simulink model "Sistema_real_NL_Din_residual"  (R2023b)
settings: Solver=VariableStepAuto  StartTime=0.0  StopTime=10.0  RelTol=1e-3
values from neighbouring files (symbols this model uses):
  alpha_cu = 3.9*10^-3    (= 0.0039)    [polos_y_ceros.m]    (also in var1.m)
  b_eq = b_m + b_l/(r^2)    (= 2.19444444444e-05)    [polos_y_ceros.m]    (also in var1.m)
  C_ts = 0.818    [polos_y_ceros.m]    (also in var1.m)
  J_eq = J_m + J_l/(r^2)    (= 1.97847222222e-05)    [polos_y_ceros.m]    (also in var1.m = 4.58263888889e-05)
  k_l = m * L_cm + m_l * L_l    (= 0.25)    [polos_y_ceros.m]    (also in var1.m = 1)
  L_d = 6.6 * 10^(-3)    (= 0.0066)    [polos_y_ceros.m]    (also in var1.m)
  L_ls = 0.8 * 10^(-3)    (= 0.0008)    [polos_y_ceros.m]    (also in var1.m)
  L_q = 5.8 * 10^(-3)    (= 0.0058)    [polos_y_ceros.m]    (also in var1.m)
  lambda_m = 0.016    [polos_y_ceros.m]    (also in var1.m)
  P_p = 3    [polos_y_ceros.m]    (also in var1.m)
  r = 120/1    (= 120)    [polos_y_ceros.m]    (also in var1.m)
  R_sREF = 1.02    [polos_y_ceros.m]    (also in var1.m)
  R_ts_amb = 146.7    [polos_y_ceros.m]    (also in var1.m)
undefined symbols (not defined in the file or in its folder): magnitude
settings Model: Creator=tomas  LastModifiedBy=tomas

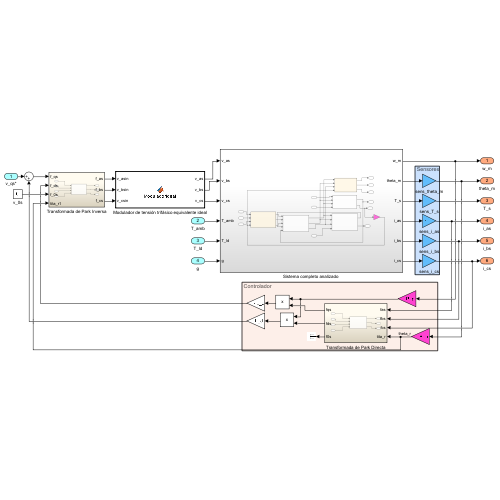
[thumbnail: Simulink's stored preview of the top-level diagram]
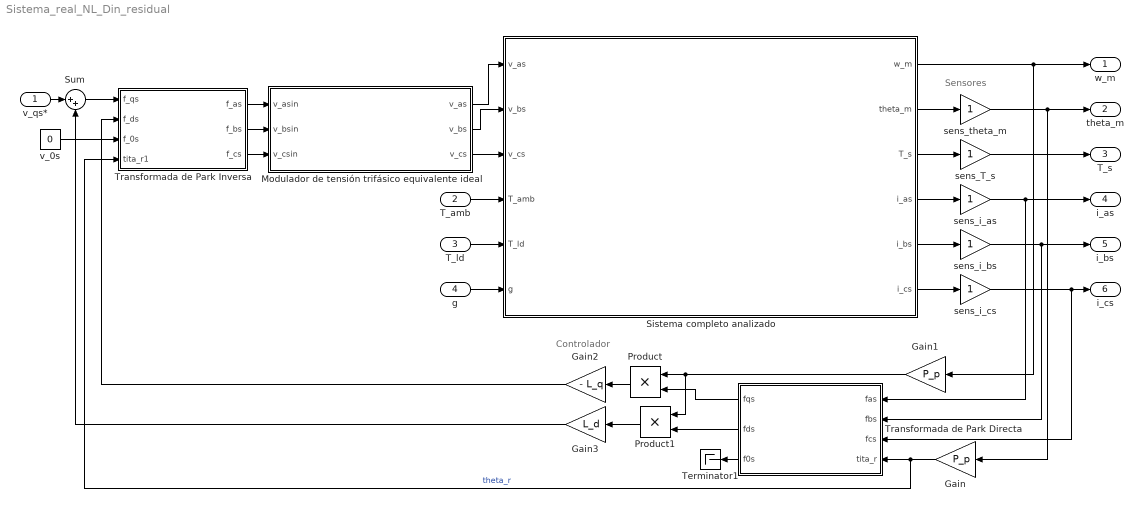
== system Sistema_real_NL_Din_residual ==
  note: Controlador
  note: Sensores
  v_qs* : Inport
  T_amb : Inport  Port=2
  T_ld : Inport  Port=3
  g : Inport  Port=4
  Gain : Gain  Gain=P_p
  Gain1 : Gain  Gain=P_p
  Gain2 : Gain  Gain=- L_q
  Gain3 : Gain  Gain=L_d
  Modulador de tensión trifásico equivalente ideal : MATLAB Function  TreatAsAtomicUnit=on
  Product : Product
  Product1 : Product
  "Sistema completo analizado " : Subsystem
  Sum : Sum  Inputs=|++
  Terminator1 : Terminator
  Transformada de Park Directa : Subsystem
  Transformada de Park Inversa : Subsystem
  sens_T_s : Gain
  sens_i_as : Gain
  sens_i_bs : Gain
  sens_i_cs : Gain
  sens_theta_m : Gain
  v_0s : Constant  Value=0
  w_m : Outport
  theta_m : Outport  Port=2
  T_s : Outport  Port=3
  i_as : Outport  Port=4
  i_bs : Outport  Port=5
  i_cs : Outport  Port=6
  wires:
  Transformada de Park Directa/3(f0s) -> Terminator1/1
  Transformada de Park Directa/2(fds) -> Product1/2
  T_ld/1 -> "Sistema completo analizado "/5(T_ld)
  Transformada de Park Inversa/3(f_cs) -> Modulador de tensión trifásico equivalente ideal/3(v_csin)
  Transformada de Park Inversa/1(f_as) -> Modulador de tensión trifásico equivalente ideal/1(v_asin)
  Transformada de Park Inversa/2(f_bs) -> Modulador de tensión trifásico equivalente ideal/2(v_bsin)
  "Sistema completo analizado "/6(i_cs) -> sens_i_cs/1
  Product/1 -> Gain2/1
  sens_i_bs/1 -> Transformada de Park Directa/2(fbs), i_bs/1
  Modulador de tensión trifásico equivalente ideal/1(v_as) -> "Sistema completo analizado "/1(v_as)
  v_0s/1 -> Transformada de Park Inversa/3(f_0s)
  "Sistema completo analizado "/4(i_as) -> sens_i_as/1
  Gain/1 -> Transformada de Park Inversa/4(tita_r1), Transformada de Park Directa/4(tita_r)  "theta_r"
  Transformada de Park Directa/1(fqs) -> Product/2
  sens_T_s/1 -> T_s/1
  "Sistema completo analizado "/3(T_s) -> sens_T_s/1
  "Sistema completo analizado "/2(theta_m) -> sens_theta_m/1
  "Sistema completo analizado "/5(i_bs) -> sens_i_bs/1
  Modulador de tensión trifásico equivalente ideal/3(v_cs) -> "Sistema completo analizado "/3(v_cs)
  Modulador de tensión trifásico equivalente ideal/2(v_bs) -> "Sistema completo analizado "/2(v_bs)
  sens_i_cs/1 -> Transformada de Park Directa/3(fcs), i_cs/1
  T_amb/1 -> "Sistema completo analizado "/4(T_amb)
  Gain2/1 -> Transformada de Park Inversa/2(f_ds)
  sens_i_as/1 -> Transformada de Park Directa/1(fas), i_as/1
  "Sistema completo analizado "/1(w_m) -> Gain1/1, w_m/1
  Gain1/1 -> Product1/1, Product/1
  sens_theta_m/1 -> Gain/1, theta_m/1
  Product1/1 -> Gain3/1
  Gain3/1 -> Sum/2
  v_qs*/1 -> Sum/1
  Sum/1 -> Transformada de Park Inversa/1(f_qs)
  g/1 -> "Sistema completo analizado "/6(g)

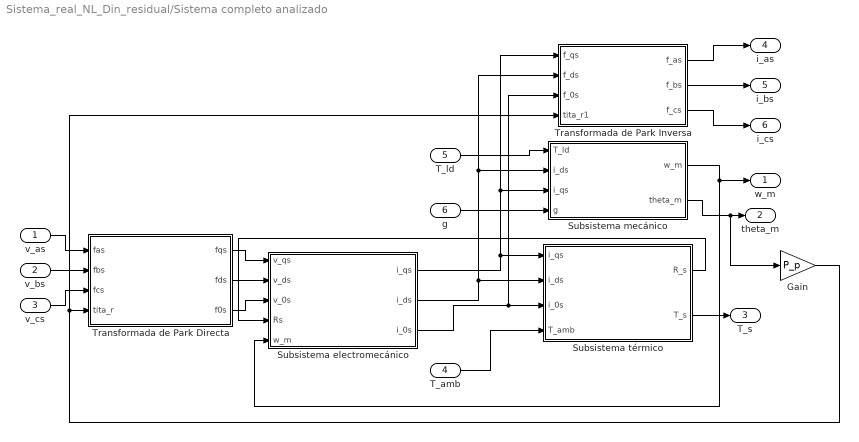
== system Sistema_real_NL_Din_residual/Sistema completo analizado  ==
  v_as : Inport
  v_bs : Inport  Port=2
  v_cs : Inport  Port=3
  T_amb : Inport  Port=4
  T_ld : Inport  Port=5
  g : Inport  Port=6
  Gain : Gain  Gain=P_p
  Subsistema electromecánico : Subsystem
  Subsistema mecánico : Subsystem
  Subsistema térmico : Subsystem
  Transformada de Park Directa : Subsystem
  Transformada de Park Inversa : Subsystem
  w_m : Outport
  theta_m : Outport  Port=2
  T_s : Outport  Port=3
  i_as : Outport  Port=4
  i_bs : Outport  Port=5
  i_cs : Outport  Port=6
  wires:
  Transformada de Park Inversa/3(f_cs) -> i_cs/1
  Subsistema mecánico/1(w_m) -> w_m/1, Subsistema electromecánico/5(w_m)
  Subsistema electromecánico/3(i_0s) -> Transformada de Park Inversa/3(f_0s), Subsistema térmico/3(i_0s)
  Transformada de Park Directa/1(fqs) -> Subsistema electromecánico/1(v_qs)
  Subsistema térmico/2(T_s) -> T_s/1
  Transformada de Park Directa/3(f0s) -> Subsistema electromecánico/3(v_0s)
  Subsistema electromecánico/2(i_ds) -> Transformada de Park Inversa/2(f_ds), Subsistema mecánico/2(i_ds), Subsistema térmico/2(i_ds)
  Gain/1 -> Transformada de Park Inversa/4(tita_r1), Transformada de Park Directa/4(tita_r)
  T_ld/1 -> Subsistema mecánico/1(T_ld)
  Transformada de Park Directa/2(fds) -> Subsistema electromecánico/2(v_ds)
  Transformada de Park Inversa/2(f_bs) -> i_bs/1
  v_bs/1 -> Transformada de Park Directa/2(fbs)
  T_amb/1 -> Subsistema térmico/4(T_amb)
  Transformada de Park Inversa/1(f_as) -> i_as/1
  v_as/1 -> Transformada de Park Directa/1(fas)
  Subsistema mecánico/2(theta_m) -> Gain/1, theta_m/1
  v_cs/1 -> Transformada de Park Directa/3(fcs)
  Subsistema electromecánico/1(i_qs) -> Transformada de Park Inversa/1(f_qs), Subsistema mecánico/3(i_qs), Subsistema térmico/1(i_qs)
  Subsistema térmico/1(R_s) -> Subsistema electromecánico/4(Rs)
  g/1 -> Subsistema mecánico/4(g)

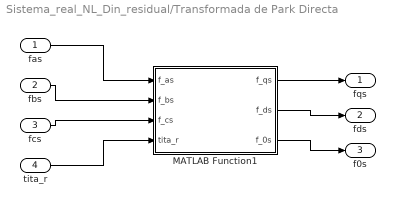
== system Sistema_real_NL_Din_residual/Transformada de Park Directa ==
  fas : Inport
  fbs : Inport  Port=2
  fcs : Inport  Port=3
  tita_r : Inport  Port=4
  MATLAB Function1 : MATLAB Function  TreatAsAtomicUnit=on
  fqs : Outport
  fds : Outport  Port=2
  f0s : Outport  Port=3
  wires:
  fas/1 -> MATLAB Function1/1(f_as)
  MATLAB Function1/3(f_0s) -> f0s/1
  MATLAB Function1/2(f_ds) -> fds/1
  fbs/1 -> MATLAB Function1/2(f_bs)
  fcs/1 -> MATLAB Function1/3(f_cs)
  tita_r/1 -> MATLAB Function1/4(tita_r)
  MATLAB Function1/1(f_qs) -> fqs/1

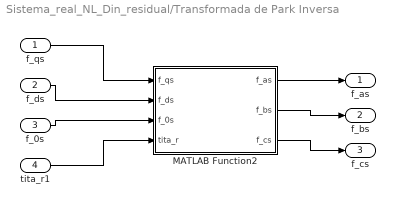
== system Sistema_real_NL_Din_residual/Transformada de Park Inversa ==
  f_qs : Inport
  f_ds : Inport  Port=2
  f_0s : Inport  Port=3
  tita_r1 : Inport  Port=4
  MATLAB Function2 : MATLAB Function  TreatAsAtomicUnit=on
  f_as : Outport
  f_bs : Outport  Port=2
  f_cs : Outport  Port=3
  wires:
  tita_r1/1 -> MATLAB Function2/4(tita_r)
  MATLAB Function2/2(f_bs) -> f_bs/1
  MATLAB Function2/1(f_as) -> f_as/1
  f_ds/1 -> MATLAB Function2/2(f_ds)
  MATLAB Function2/3(f_cs) -> f_cs/1
  f_0s/1 -> MATLAB Function2/3(f_0s)
  f_qs/1 -> MATLAB Function2/1(f_qs)

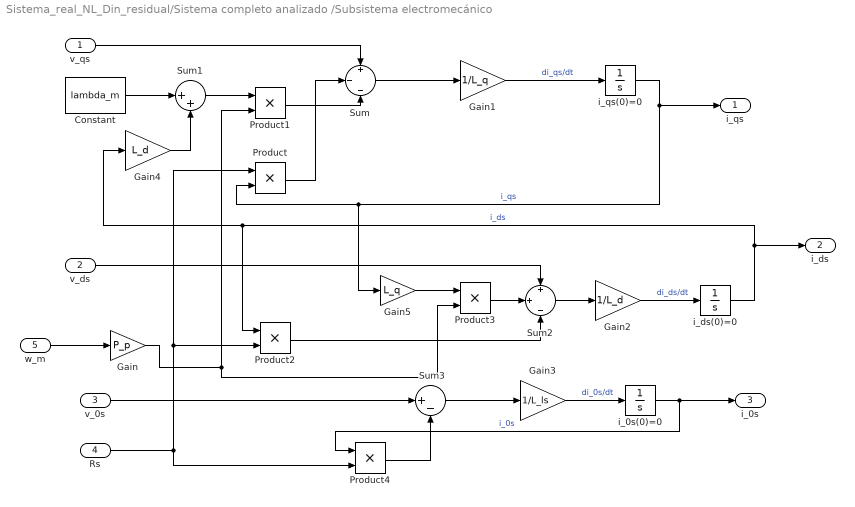
== system Sistema_real_NL_Din_residual/Sistema completo analizado /Subsistema electromecánico ==
  v_qs : Inport
  v_ds : Inport  Port=2
  v_0s : Inport  Port=3
  Rs : Inport  Port=4
  w_m : Inport  Port=5
  Constant : Constant  Value=lambda_m
  Gain : Gain  Gain=P_p
  Gain1 : Gain  Gain=1/L_q
  Gain2 : Gain  Gain=1/L_d
  Gain3 : Gain  Gain=1/L_ls
  Gain4 : Gain  Gain=L_d
  Gain5 : Gain  Gain=L_q
  Product{,1..4} (5 alike) : Product
  Sum : Sum  Inputs=+|-|-
  Sum1 : Sum  Inputs=|++
  Sum2 : Sum  Inputs=+|+|-
  Sum3 : Sum  Inputs=|+-
  i_0s(0)=0 : Integrator
  i_ds(0)=0 : Integrator
  i_qs(0)=0 : Integrator
  i_qs : Outport
  i_ds : Outport  Port=2
  i_0s : Outport  Port=3
  wires:
  Gain1/1 -> i_qs(0)=0/1  "di_qs/dt"
  Rs/1 -> Product2/2, Product/1, Product4/2
  i_qs(0)=0/1 -> Gain5/1, Product/2, i_qs/1  "i_qs"
  Sum2/1 -> Gain2/1
  Product1/1 -> Sum/3
  Product4/1 -> Sum3/2
  v_0s/1 -> Sum3/1
  Product3/1 -> Sum2/2
  Gain3/1 -> i_0s(0)=0/1  "di_0s/dt"
  Gain/1 -> Product3/2, Product1/2
  v_qs/1 -> Sum/1
  Sum1/1 -> Product1/1
  Gain5/1 -> Product3/1
  Sum3/1 -> Gain3/1
  i_0s(0)=0/1 -> Product4/1, i_0s/1  "i_0s"
  Product2/1 -> Sum2/3
  Gain2/1 -> i_ds(0)=0/1  "di_ds/dt"
  Constant/1 -> Sum1/1
  Gain4/1 -> Sum1/2
  Sum/1 -> Gain1/1
  Product/1 -> Sum/2
  w_m/1 -> Gain/1
  i_ds(0)=0/1 -> Product2/1, Gain4/1, i_ds/1  "i_ds"
  v_ds/1 -> Sum2/1

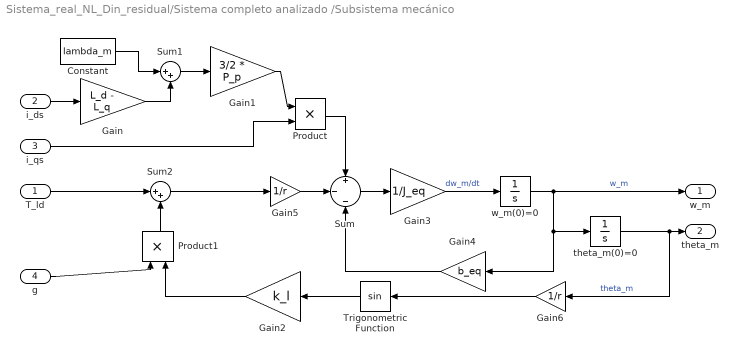
== system Sistema_real_NL_Din_residual/Sistema completo analizado /Subsistema mecánico ==
  T_ld : Inport
  i_ds : Inport  Port=2
  i_qs : Inport  Port=3
  g : Inport  Port=4
  Constant : Constant  Value=lambda_m
  Gain : Gain  Gain=L_d - L_q
  Gain1 : Gain  Gain=3/2 * P_p
  Gain2 : Gain  Gain=k_l
  Gain3 : Gain  Gain=1/J_eq
  Gain4 : Gain  Gain=b_eq
  Gain5 : Gain  Gain=1/r
  Gain6 : Gain  Gain=1/r
  Product : Product
  Product1 : Product
  Sum : Sum  Inputs=+|-|-
  Sum1 : Sum  Inputs=|++
  Sum2 : Sum  Inputs=|++
  Trigonometric Function : Trigonometry
  theta_m(0)=0 : Integrator
  w_m(0)=0 : Integrator
  w_m : Outport
  theta_m : Outport  Port=2
  wires:
  w_m(0)=0/1 -> w_m/1, theta_m(0)=0/1, Gain4/1  "w_m"
  Sum/1 -> Gain3/1
  Gain3/1 -> w_m(0)=0/1  "dw_m/dt"
  i_ds/1 -> Gain/1
  Constant/1 -> Sum1/1
  Gain/1 -> Sum1/2
  Sum1/1 -> Gain1/1
  Gain1/1 -> Product/1
  i_qs/1 -> Product/2
  Product/1 -> Sum/1
  Gain4/1 -> Sum/3
  Gain5/1 -> Sum/2
  Trigonometric Function/1 -> Gain2/1
  Gain2/1 -> Product1/2
  theta_m(0)=0/1 -> Gain6/1, theta_m/1  "theta_m"
  T_ld/1 -> Sum2/1
  Sum2/1 -> Gain5/1
  Gain6/1 -> Trigonometric Function/1
  g/1 -> Product1/1
  Product1/1 -> Sum2/2

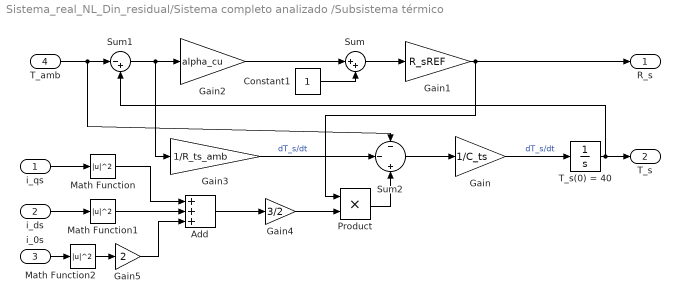
== system Sistema_real_NL_Din_residual/Sistema completo analizado /Subsistema térmico ==
  i_qs : Inport
  i_ds : Inport  Port=2
  i_0s : Inport  Port=3
  T_amb : Inport  Port=4
  Add : Sum  Inputs=+++
  Constant1 : Constant
  Gain : Gain  Gain=1/C_ts
  Gain1 : Gain  Gain=R_sREF
  Gain2 : Gain  Gain=alpha_cu
  Gain3 : Gain  Gain=1/R_ts_amb
  Gain4 : Gain  Gain=3/2
  Gain5 : Gain  Gain=2
  Math Function : Math  Operator=magnitude^2
  Math Function1 : Math  Operator=magnitude^2
  Math Function2 : Math  Operator=magnitude^2
  Product : Product
  Sum : Sum  Inputs=|++
  Sum1 : Sum  Inputs=|-+
  Sum2 : Sum  Inputs=-|-|+
  T_s(0) = 40 : Integrator  InitialCondition=40
  R_s : Outport
  T_s : Outport  Port=2
  wires:
  Math Function2/1 -> Gain5/1
  Gain3/1 -> Sum2/2  "dT_s/dt"
  Math Function/1 -> Add/1
  T_amb/1 -> Sum2/1, Sum1/1
  Sum2/1 -> Gain/1
  Sum/1 -> Gain1/1
  Gain2/1 -> Sum/1
  Gain1/1 -> Product/1, R_s/1
  Product/1 -> Sum2/3
  i_ds/1 -> Math Function1/1
  Gain/1 -> T_s(0) = 40/1  "dT_s/dt"
  Constant1/1 -> Sum/2
  Gain4/1 -> Product/2
  T_s(0) = 40/1 -> T_s/1, Sum1/2
  Math Function1/1 -> Add/2
  i_0s/1 -> Math Function2/1
  Sum1/1 -> Gain3/1, Gain2/1
  Add/1 -> Gain4/1
  Gain5/1 -> Add/3
  i_qs/1 -> Math Function/1

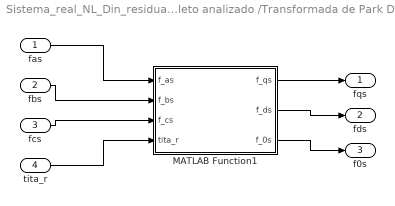
== system Sistema_real_NL_Din_residual/Sistema completo analizado /Transformada de Park Directa ==
  fas : Inport
  fbs : Inport  Port=2
  fcs : Inport  Port=3
  tita_r : Inport  Port=4
  MATLAB Function1 : MATLAB Function  TreatAsAtomicUnit=on
  fqs : Outport
  fds : Outport  Port=2
  f0s : Outport  Port=3
  wires:
  fas/1 -> MATLAB Function1/1(f_as)
  MATLAB Function1/3(f_0s) -> f0s/1
  MATLAB Function1/2(f_ds) -> fds/1
  fbs/1 -> MATLAB Function1/2(f_bs)
  fcs/1 -> MATLAB Function1/3(f_cs)
  tita_r/1 -> MATLAB Function1/4(tita_r)
  MATLAB Function1/1(f_qs) -> fqs/1

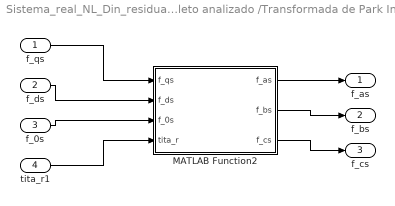
== system Sistema_real_NL_Din_residual/Sistema completo analizado /Transformada de Park Inversa ==
  f_qs : Inport
  f_ds : Inport  Port=2
  f_0s : Inport  Port=3
  tita_r1 : Inport  Port=4
  MATLAB Function2 : MATLAB Function  TreatAsAtomicUnit=on
  f_as : Outport
  f_bs : Outport  Port=2
  f_cs : Outport  Port=3
  wires:
  tita_r1/1 -> MATLAB Function2/4(tita_r)
  MATLAB Function2/2(f_bs) -> f_bs/1
  MATLAB Function2/1(f_as) -> f_as/1
  f_ds/1 -> MATLAB Function2/2(f_ds)
  MATLAB Function2/3(f_cs) -> f_cs/1
  f_0s/1 -> MATLAB Function2/3(f_0s)
  f_qs/1 -> MATLAB Function2/1(f_qs)

== matlab function Sistema_real_NL_Din_residual/Sistema completo analizado /Transformada de Park Directa/MATLAB Function1 ==
  data: f_as input; f_qs output; f_bs input; f_cs input; tita_r input; f_ds output; f_0s output
function [f_qs, f_ds, f_0s] = parkDir(f_as,f_bs,f_cs,tita_r)

answer = 2/3 * [cos(tita_r), cos(tita_r - 2*pi/3), cos(tita_r + 2*pi/3);
         sin(tita_r), sin(tita_r - 2*pi/3), sin(tita_r + 2*pi/3);
         1/2, 1/2, 1/2] * [f_as;f_bs;f_cs];

f_qs = answer(1);
f_ds = answer(2);
f_0s = answer(3);

== matlab function Sistema_real_NL_Din_residual/Transformada de Park Directa/MATLAB Function1 ==
  data: f_as input; f_qs output; f_bs input; f_cs input; tita_r input; f_ds output; f_0s output
function [f_qs, f_ds, f_0s] = parkDir(f_as,f_bs,f_cs,tita_r)

answer = 2/3 * [cos(tita_r), cos(tita_r - 2*pi/3), cos(tita_r + 2*pi/3);
         sin(tita_r), sin(tita_r - 2*pi/3), sin(tita_r + 2*pi/3);
         1/2, 1/2, 1/2] * [f_as;f_bs;f_cs];

f_qs = answer(1);
f_ds = answer(2);
f_0s = answer(3);

== matlab function Sistema_real_NL_Din_residual/Sistema completo analizado /Transformada de Park Inversa/MATLAB Function2 ==
  data: f_qs input; f_as output; f_ds input; f_0s input; tita_r input; f_bs output; f_cs output
function [f_as, f_bs, f_cs] = parkInv(f_qs,f_ds,f_0s,tita_r)

answer = [cos(tita_r), sin(tita_r), 1;
         cos(tita_r - 2*pi/3), sin(tita_r - 2*pi/3), 1;
         cos(tita_r + 2*pi/3), sin(tita_r + 2*pi/3), 1] * [f_qs;f_ds;f_0s]; 

f_as = answer(1);
f_bs = answer(2);
f_cs = answer(3);

== matlab function Sistema_real_NL_Din_residual/Modulador de tensión trifásico equivalente ideal ==
  data: v_asin input; v_as output; v_bsin input; v_csin input; v_bs output; v_cs output
function [v_as,v_bs,v_cs] = ModuladorIdeal(v_asin,v_bsin, v_csin)
v_as=v_asin;
v_bs=v_bsin;
v_cs=v_csin;

== matlab function Sistema_real_NL_Din_residual/Transformada de Park Inversa/MATLAB Function2 ==
  data: f_qs input; f_as output; f_ds input; f_0s input; tita_r input; f_bs output; f_cs output
function [f_as, f_bs, f_cs] = parkInv(f_qs,f_ds,f_0s,tita_r)

answer = [cos(tita_r), sin(tita_r), 1;
         cos(tita_r - 2*pi/3), sin(tita_r - 2*pi/3), 1;
         cos(tita_r + 2*pi/3), sin(tita_r + 2*pi/3), 1] * [f_qs;f_ds;f_0s]; 

f_as = answer(1);
f_bs = answer(2);
f_cs = answer(3);
